simulink model "pdmTransmissionCasing3_new"  (R2020b)
settings: Solver=VariableStepAuto  StartTime=0.0  StopTime=50  FixedStep=0.1  MaxStep=1e-1  RelTol=1e-1  AbsTol=1e-1  EnableMultiTasking=on
PreLoadFcn:
  | ClutchRadius = 100;
  | DampingCoeff = 0.1;
  | SGain = 1;
  | ShaftWear = 0;
  | ToothFaultGain = 0;
  | SDrift = 0;
undefined symbols (not defined in the file or in its folder): sigbuilder_block
libraries: fl_lib x42, nesl_utility x22, sdl_lib x6, commchan3 x2
(part 1 of 2)
CloseFcn:
  | try,close(h1_sdl_transmission_2spd),end
  | clear h1_sdl_transmission_2spd
  | 
  | 
  | clear simlog_sdl_transmission_2spd
  | clear logsout_sdl_transmission_2spd
Description:
  | Two-Speed Transmission
settings Model: FPTRunName=Active  ExtModeAutoUpdateStatusClock=off  Creator=The MathWorks, Inc.  LastModifiedBy=hubert
settings SolverCC: AutoScaleAbsTol=off
settings DataIOCC: MaxDataPoints=10000  SaveFinalState=on  SaveFormat=StructureWithTime  SaveOutput=off  SaveState=on  SaveTime=off  ReturnWorkspaceOutputs=off  LoggingToFile=on  LoggingFileName=out
settings OptimizationCC: ExpressionDepthLimit=2147483647  InitFltsAndDblsToZero=on  LifeSpan=inf
settings DebuggingCC: AlgebraicLoopMsg=none  SaveWithParameterizedLinksMsg=none  UnderspecifiedInitializationDetection=Classic  MergeDetectMultiDrivingBlocksExec=none  CheckExecutionContextPreStartOutputMsg=on  CheckExecutionContextRuntimeOutputMsg=on  SignalResolutionControl=TryResolveAllWithWarning  MultiTaskDSMMsg=warning  MultiTaskCondExecSysMsg=none  FcnCallInpInsideContextMsg=warning  StateNameClashWarn=warning  SFUnexpectedBacktrackingDiag=warning  SFNoUnconditionalDefaultTransitionDiag=warning  SFExecutionAtInitializationDiag=none  ArithmeticOperatorsInVariantConditions=warning
settings HardwareCC: ProdBitPerPointer=32  ProdBitPerSizeT=32  ProdBitPerPtrDiffT=32  ProdLargestAtomicFloat=None  ProdIntDivRoundTo=Undefined  ProdEndianess=Unspecified  ProdWordSize=32  ProdHWDeviceType=32-bit Generic  TargetBitPerLong=64  TargetBitPerPointer=64  TargetBitPerSizeT=64  TargetBitPerPtrDiffT=64  TargetLongLongMode=on  TargetIntDivRoundTo=Zero  TargetEndianess=LittleEndian  TargetWordSize=64  TargetHWDeviceType=MATLAB Host  ProdEqTarget=off
settings ModelReferenceCC: UpdateModelReferenceTargets=IfOutOfDate  PropagateSignalLabelsOutOfModel=off
settings SFSimCC: SimUseLocalCustomCode=off  CustomCodeUndefinedFunction=UseInterfaceOnly
settings RTWCC: RTWUseLocalCustomCode=off
settings CodeAppCC: StateflowObjectComments=on
settings GRTTargetCC: TargetLangStandard=C89/C90 (ANSI)  CombineOutputUpdateFcns=off  GRTInterface=on
settings ConfigComp: CovMetricSettings=dw  CovSaveCumulativeToWorkspaceVar=on  CovSaveSingleToWorkspaceVar=on  CovExternalEMLEnable=off
settings SimscapeCC: SimscapeNormalizeSystem=off  SimscapeLogName=simlog_sdl_transmission_2spd  SimscapeLogDataHistory=10000

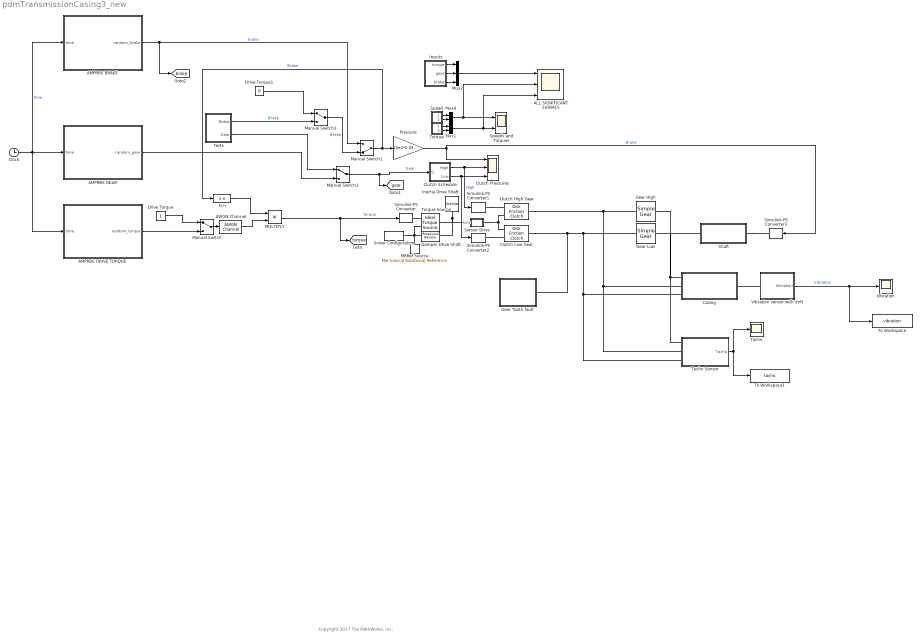
== system pdmTransmissionCasing3_new ==
  note: Copyright 2017 The MathWorks, Inc.
  ALL SIGNIFICANT SIGNALS : Scope  NumInputPorts=3
  AMPRBS BRAKE : Subsystem
  AMPRBS DRIVE TORQUE : Subsystem
  AMPRBS GEAR : Subsystem
  AWGN Channel : commchan3/AWGN Channel  InputProcessing=Columns as channels (frame based)  seed=67  noiseMode=Variance from mask  EbNodB=10  EsNodB=10  SNRdB=10  bitsPerSym=1  Ps=1  Tsym=0.1  variance=0.001
  Casing : Subsystem
  Clock : Clock
  Clutch High Gear : sdl_lib/Clutches/Disk Friction Clutch  geometry_model=1  r_eff=100 mm  d_o=150 mm  d_i=100 mm  nS=4  piston_area=0.001 m^2  unidirectional=0  friction_model=1  mu_w_vector=[ 0 0.1 0.2 0.3 0.4 0.5 1 2 5 10 100 1000 ] rad/s  temperature_TLU=[280.0, 300.0, 320.0] K  mu_static=0.35  mu_static_vector=[0.4, 0.38, 0.36]  mu_coulomb=0.3  mu_coulomb_vector=[ 0.29 0.28 0.26 0.22 0.21 0.2 0.2 0.19 0.19 0.19 0.19 0.19 ]  mu_coulomb_temp_vector=[0.3, 0.28, 0.25]  mu_coulomb_matrix=[0.34, 0.32, 0.3; 0.3, 0.28, 0.25; 0.25, 0.2, 0.15]  mu_interp_method=1  mu_extrap_method=1  d_f=1  w_tol=0.001 rad/s  pressure_min=100 Pa  mu_visc=0 N*m/(rad/s)  initial_state_locked=0  enable_faults=simscape.enum.onoff.off  fault_type=sdl.enum.clutchFault.lock  external_fault=simscape.enum.onoff.off  temporal_fault=simscape.enum.onoff.off  fault_time=5 s  report_fault=simscape.enum.assert.action.none  thermal_mass=25 kJ/K  T_init=300 K
      settings: SourceProductName=Driveline  InternalSimscapePortConfiguration="{\"Bottom\":[],\"Left\":[{\"id\":\"P\",\"label\":\"P\",\"type\":\"input\"},{\"id\":\"B\",\"label\":\"B\",\"type\":\"foundation.mechanical.rotational.rotational\"}],\"Right\":[{\"id\":\"F\",\"label\":\"F\",\"type\":\"foundation.mechanical.rotational.rotational\"}],\"Top\":[]}"
  Clutch Low Gear : sdl_lib/Clutches/Disk Friction Clutch  geometry_model=1  r_eff=ClutchRadius mm  d_o=150 mm  d_i=100 mm  nS=4  piston_area=0.001 m^2  unidirectional=0  friction_model=1  mu_w_vector=[ 0 0.1 0.2 0.3 0.4 0.5 1 2 5 10 100 1000 ] rad/s  temperature_TLU=[280.0, 300.0, 320.0] K  mu_static=0.35  mu_static_vector=[0.4, 0.38, 0.36]  mu_coulomb=0.3  mu_coulomb_vector=[ 0.29 0.28 0.26 0.22 0.21 0.2 0.2 0.19 0.19 0.19 0.19 0.19 ]  mu_coulomb_temp_vector=[0.3, 0.28, 0.25]  mu_coulomb_matrix=[0.34, 0.32, 0.3; 0.3, 0.28, 0.25; 0.25, 0.2, 0.15]  mu_interp_method=1  mu_extrap_method=1  d_f=1  w_tol=0.001 rad/s  pressure_min=100 Pa  mu_visc=0 N*m/(rad/s)  initial_state_locked=0  enable_faults=simscape.enum.onoff.off  fault_type=sdl.enum.clutchFault.lock  external_fault=simscape.enum.onoff.off  temporal_fault=simscape.enum.onoff.off  fault_time=5 s  report_fault=simscape.enum.assert.action.none  thermal_mass=25 kJ/K  T_init=300 K
      settings: SourceProductName=Driveline  InternalSimscapePortConfiguration="{\"Bottom\":[],\"Left\":[{\"id\":\"P\",\"label\":\"P\",\"type\":\"input\"},{\"id\":\"B\",\"label\":\"B\",\"type\":\"foundation.mechanical.rotational.rotational\"}],\"Right\":[{\"id\":\"F\",\"label\":\"F\",\"type\":\"foundation.mechanical.rotational.rotational\"}],\"Top\":[]}"
  Clutch Pressures : Scope  NumInputPorts=3
  Clutch Schedule : Subsystem
  Damper Drive Shaft : fl_lib/Mechanical/Rotational Elements/Rotational Damper  D=DampingCoeff N*m/(rad/s)  w_specify=off  w_priority=High  w=0 rad/s  w_nominal_specify=off  w_nominal_unit=rad/s  w_nominal_value=1  t_specify=off  t_priority=High  t=0 N*m  t_nominal_specify=off  t_nominal_unit=N*m  t_nominal_value=1
      settings: SourceProductName=Foundation Library
  Drive Torque : Constant
  Drive Torque1 : Constant  Value=0
  Fcn : Fcn  Expr=1-u
  Gear High : sdl_lib/Gears/Simple Gear  ratio=2  rotation_direction=3-2*(2)  friction_model=1  mu_visc=[ 0 0 ] N*m/(rad/s)  T_noload=0.1 N*m  T_nom=5 N*m  efficiency_nom=0.8  efficiency=0.8  temperature_TLU=[ 280 300 320 ] K  load_TLU=[ 1 5 10 ] N*m  efficiency_TLU=[ 0.95 0.9 0.85 ]  efficiency_TLU2=[ 0.85 0.8 0.75; 0.95 0.9 0.85; 0.85 0.8 0.7 ]  w_thr=0.01 rad/s  pwr_thr=0.001 W  thermal_mass=50 J/K  enable_faults=simscape.enum.onoff.off  efficiency_fault=0.05  external_fault=simscape.enum.onoff.off  temporal_fault=simscape.enum.onoff.off  fault_time=5 s  fault_angles=pi / 12 rad  report_fault=(1)-1  temperature_specify=off  temperature_priority=High  temperature=300 K  temperature_nominal_specify=off  temperature_nominal_unit=K  temperature_nominal_value=1
      settings: SourceProductName=Driveline
  Gear Low : sdl_lib/Gears/Simple Gear  ratio=5  rotation_direction=3-2*(2)  friction_model=1  mu_visc=[ 0 0 ] N*m/(rad/s)  T_noload=0.1 N*m  T_nom=5 N*m  efficiency_nom=0.8  efficiency=0.8  temperature_TLU=[ 280 300 320 ] K  load_TLU=[ 1 5 10 ] N*m  efficiency_TLU=[ 0.95 0.9 0.85 ]  efficiency_TLU2=[ 0.85 0.8 0.75; 0.95 0.9 0.85; 0.85 0.8 0.7 ]  w_thr=0.01 rad/s  pwr_thr=0.001 W  thermal_mass=50 J/K  enable_faults=simscape.enum.onoff.off  efficiency_fault=0.05  external_fault=simscape.enum.onoff.off  temporal_fault=simscape.enum.onoff.off  fault_time=5 s  fault_angles=pi / 12 rad  report_fault=(1)-1  temperature_specify=off  temperature_priority=High  temperature=300 K  temperature_nominal_specify=off  temperature_nominal_unit=K  temperature_nominal_value=1
      settings: SourceProductName=Driveline
  Gear Tooth fault : Subsystem
  Inertia Drive Shaft : fl_lib/Mechanical/Rotational Elements/Inertia  inertia=1*0.01 kg*m^2  num_ports=foundation.enum.numPorts2.one  w_specify=off  w_priority=High  w=0 rad/s  w_nominal_specify=off  w_nominal_unit=rad/s  w_nominal_value=1  t_specify=off  t_priority=High  t=0 N*m  t_nominal_specify=off  t_nominal_unit=N*m  t_nominal_value=1
      settings: SourceProductName=Foundation Library
  Inputs : Subsystem
  MRRef Source : fl_lib/Mechanical/Rotational Elements/Mechanical Rotational Reference
      settings: SourceProductName=Foundation Library
  MULTIPLY : Product  Inputs=**
  Manual Switch : ManualSwitch
  Manual Switch1 : ManualSwitch  CurrentSetting=0
  Manual Switch2 : ManualSwitch
  Manual Switch3 : ManualSwitch
  Mux1 : Mux  Inputs=2
  Mux2 : Mux  Inputs=3
  Mux4 : Mux  Inputs=2
  Pressure : Gain  Gain=10e2*0.03  SaturateOnIntegerOverflow=on  OutDataTypeStr=Inherit: Same as input  ParamDataTypeStr=Inherit: Same as input
  Sensor Drive : Subsystem
      mask Display: disp('SD')
  Shaft : Subsystem  Variant=on
  Simulink-PS Converter : nesl_utility/Simulink-PS Converter  PhysicalDomain=network_engine_domain  SubClassName=ps_input  LeftPortType=input  RightPortType=output  PseudoPeriodic=off  Frequencies=[]  NoiseDistribution=none  NoiseParameters=[]  Unit=1  AffineConversion=off  FilteringAndDerivatives=zero  SimscapeFilterOrder=1  InputFilterTimeConstant=.001  UdotUserProvided=0
      settings: SourceProductName=Utilities
  Simulink-PS Converter1 : nesl_utility/Simulink-PS Converter  PhysicalDomain=network_engine_domain  SubClassName=ps_input  LeftPortType=input  RightPortType=output  PseudoPeriodic=off  Frequencies=[]  NoiseDistribution=none  NoiseParameters=[]  Unit=Pa  AffineConversion=off  FilteringAndDerivatives=zero  SimscapeFilterOrder=1  InputFilterTimeConstant=.001  UdotUserProvided=0
      settings: SourceProductName=Utilities
  Simulink-PS Converter2 : nesl_utility/Simulink-PS Converter  PhysicalDomain=network_engine_domain  SubClassName=ps_input  LeftPortType=input  RightPortType=output  PseudoPeriodic=off  Frequencies=[]  NoiseDistribution=none  NoiseParameters=[]  Unit=Pa  AffineConversion=off  FilteringAndDerivatives=zero  SimscapeFilterOrder=1  InputFilterTimeConstant=.001  UdotUserProvided=0
      settings: SourceProductName=Utilities
  Simulink-PS Converter3 : nesl_utility/Simulink-PS Converter  PhysicalDomain=network_engine_domain  SubClassName=ps_input  LeftPortType=input  RightPortType=output  PseudoPeriodic=off  Frequencies=[]  NoiseDistribution=none  NoiseParameters=[]  Unit=Pa  AffineConversion=off  FilteringAndDerivatives=zero  SimscapeFilterOrder=1  InputFilterTimeConstant=.001  UdotUserProvided=0
      settings: SourceProductName=Utilities
  Solver Configuration : nesl_utility/Solver Configuration  PhysicalDomain=network_engine_domain  SubClassName=solver  LeftPortType=input  RightPortType=generic  Tones=[]  Harmonics=[]  SimulateNoise=off  Profile=off  UseLocalSampling=off  EnableSwitchedLinearOptims=on  FrequencyDomain=off  UseCCode=off  RelTol=0.001  AbsTol=1e-06  MinStep=1e-09  ToWorkspace=off  RevertToSquareIcSolve=off  NumHomotopyIterations=100  PhasorMode=off  PhasorModeNumHarmonics=1  DoDC=off  ResidualTolerance=1e-9  UseLocalSolver=off  LocalSolverChoice=NE_BACKWARD_EULER_ADVANCER  LocalSolverSampleTime=.001  DoFixedCost=off  MaxNonlinIter=3  MaxModeIter=2  ComputeImpulses=off  ImpulseIterations=2  LinearAlgebra=Sparse  EquationFormulation=NE_TIME_EF  DelaysMemoryBudget=1024  AutomaticFiltering=on  FilteringTimeConstant=0.001  PartitionStorageMethod=AS_NEEDED  PartitionMemoryBudget=1024  PartitionMethod=FAST
      settings: SourceProductName=Utilities
  Speed : Subsystem
  Speeds and Torques : Scope  NumInputPorts=2
  Tacho : Scope
  Tacho Sensor : Subsystem
  Tests : Subsystem  Tag=STV Subsys  LoadFcn=sigbuilder_block('load');  StartFcn=sigbuilder_block('start');  StopFcn=sigbuilder_block('stop');  ClipboardFcn=sigbuilder_block('clipboard');  mask(Sigbuilder block){tuvar=[0:10]}
      mask help: Simulink:masks:SigbuilderBlock_MD
      mask init:
      | if ~strcmp(get_param(bdroot(gcbh),'SimulationStatus'),'stopped') tuvar = sigbuilder_block('maskInit'); end
      settings: CopyFcn=sigbuilder_block('copy');  DeleteFcn=sigbuilder_block('delete');  ModelCloseFcn=sigbuilder_block('modelClose');  PreSaveFcn=sigbuilder_block('preSave');  PauseFcn=sigbuilder_block('pause');  ContinueFcn=sigbuilder_block('continue');  NameChangeFcn=sigbuilder_block('namechange');  OpenFcn=sigbuilder_block('open',[1600.5 1117.5 2958 1396.5 ]);  CloseFcn=sigbuilder_block('close');
      mask Display: plot(0, 0, 100, 100,[2, 2, 32, 32, 2], [68, 8, 8, 68, 68],[32, 2], [38, 38], [32, 19, 2],[53, 60, 44], [32, 17, 17, 2],[16, 16, 31, 31]);txt = getActiveGroup(gcbh);text(2, 100, txt,'verticalAlignment', 'top');
  To Workspace : ToWorkspace  VariableName=vibration  SaveFormat=Timeseries  SampleTime=0.1
  To Workspace1 : ToWorkspace  VariableName=tacho  SaveFormat=Timeseries  SampleTime=0.1
  Torque : Subsystem
  Torque Source : fl_lib/Mechanical/Mechanical Sources/Ideal Torque Source
      settings: SourceProductName=Foundation Library
  Vibration : Scope
  Vibration sensor with drift : Subsystem  VariantControl=Variant < 0
  tag scope: brake=global, gear=global, torque=global
  wires:
  Clutch Schedule/1(High) -> Clutch Pressures/2, Simulink-PS Converter1/1  "High"
  Clutch Schedule/2(Low) -> Clutch Pressures/3, Simulink-PS Converter2/1  "Low"
  Tests/2(Gear) -> Manual Switch2/1
  Manual Switch1/1 -> Fcn/1, Pressure/1  "Brake"
  Speed/1(wD) -> Mux4/1
  Speed/2(wO) -> Mux4/2
  Mux4/1 -> ALL SIGNIFICANT SIGNALS/2, Speeds and Torques/1
  Torque/1(tD) -> Mux1/1
  Torque/2(tO) -> Mux1/2
  Mux1/1 -> ALL SIGNIFICANT SIGNALS/3, Speeds and Torques/2
  Vibration sensor with drift/1(Vibration) -> To Workspace/1, Vibration/1  "Vibration"
  Tacho Sensor/1(Tacho) -> Tacho/1, To Workspace1/1
  Clock/1 -> AMPRBS DRIVE TORQUE/1(time), AMPRBS BRAKE/1(time), AMPRBS GEAR/1(time)  "time"
  AMPRBS BRAKE/1(random_brake) -> [brake], Manual Switch1/1  "brake"
  AMPRBS GEAR/1(random_gear) -> Manual Switch2/2
  Manual Switch2/1 -> [gear], Clutch Schedule/1(G)  "Gear"
  AMPRBS DRIVE TORQUE/1(random_torque) -> Manual Switch/2
  Fcn/1 -> MULTIPLY/1
  Manual Switch/1 -> AWGN Channel/1
  MULTIPLY/1 -> Simulink-PS Converter/1, [torque]  "torque"
  Inputs/1(torque) -> Mux2/1
  Inputs/2(gear) -> Mux2/2
  Inputs/3(brake) -> Mux2/3
  Mux2/1 -> ALL SIGNIFICANT SIGNALS/1
  Drive Torque/1 -> Manual Switch/1
  AWGN Channel/1 -> MULTIPLY/2
  Pressure/1 -> Clutch Pressures/1, Simulink-PS Converter3/1  "Brake"
  Drive Torque1/1 -> Manual Switch3/1
  Tests/1(Brake) -> Manual Switch3/2  "Brake"
  Manual Switch3/1 -> Manual Switch1/2  "Brake"
  connections:
  Clutch High Gear/RConn1 -- Tacho Sensor/LConn2 -- Casing/LConn2 -- Gear High/LConn1
  Simulink-PS Converter1/RConn1 -- Clutch High Gear/LConn1
  Clutch Low Gear/RConn1 -- Gear Tooth fault/LConn1 -- Tacho Sensor/LConn3 -- Casing/LConn3 -- Gear Low/LConn1
  Clutch High Gear/LConn2 -- Clutch Low Gear/LConn2 -- Sensor Drive/RConn1
  Simulink-PS Converter2/RConn1 -- Clutch Low Gear/LConn1
  Inertia Drive Shaft/LConn1 -- Torque Source/LConn1 -- Damper Drive Shaft/LConn1 -- Sensor Drive/LConn1
  Torque Source/RConn2 -- Damper Drive Shaft/RConn1 -- MRRef Source/LConn1 -- Solver Configuration/RConn1
  Torque Source/RConn1 -- Simulink-PS Converter/RConn1
  Vibration sensor with drift/LConn1 -- Casing/RConn1
  Shaft/LConn1 -- Gear Low/RConn1 -- Gear High/RConn1 -- Tacho Sensor/LConn1 -- Casing/LConn1
  Shaft/RConn1 -- Simulink-PS Converter3/RConn1

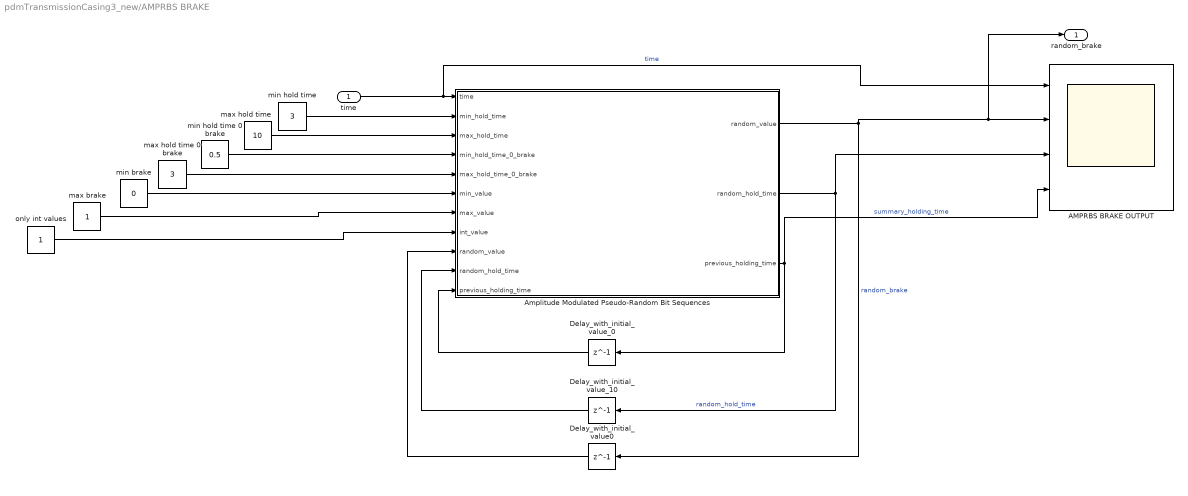
== system pdmTransmissionCasing3_new/AMPRBS BRAKE ==
  time : Inport
  AMPRBS BRAKE OUTPUT : Scope  NumInputPorts=4
  Amplitude Modulated Pseudo-Random Bit Sequences : MATLAB Function  TreatAsAtomicUnit=on  SystemSampleTime=0.1
  Delay_with_initial_value0 : Delay  DelayLength=1  InitialCondition=0
  Delay_with_initial_value_0 : Delay  DelayLength=1  InitialCondition=0
  Delay_with_initial_value_10 : Delay  DelayLength=1  InitialCondition=10
  max brake : Constant
  max hold time : Constant  Value=10
  max hold time 0 brake : Constant  Value=3
  min brake : Constant  Value=0
  min hold time : Constant  Value=3
  min hold time 0 brake : Constant  Value=0.5
  only int values : Constant
  random_brake : Outport
  wires:
  Delay_with_initial_value_10/1 -> Amplitude Modulated Pseudo-Random Bit Sequences/10("random_hold_time ")
  Amplitude Modulated Pseudo-Random Bit Sequences/1(random_value) -> random_brake/1, AMPRBS BRAKE OUTPUT/2, Delay_with_initial_value0/1  "random_brake"
  time/1 -> AMPRBS BRAKE OUTPUT/1, Amplitude Modulated Pseudo-Random Bit Sequences/1(time)  "time"
  Amplitude Modulated Pseudo-Random Bit Sequences/3(previous_holding_time) -> AMPRBS BRAKE OUTPUT/4, Delay_with_initial_value_0/1  "summary_holding_time"
  Delay_with_initial_value_0/1 -> Amplitude Modulated Pseudo-Random Bit Sequences/11("previous_holding_time ")
  Amplitude Modulated Pseudo-Random Bit Sequences/2(random_hold_time) -> AMPRBS BRAKE OUTPUT/3, Delay_with_initial_value_10/1  "random_hold_time"
  Delay_with_initial_value0/1 -> Amplitude Modulated Pseudo-Random Bit Sequences/9("random_value ")
  min brake/1 -> Amplitude Modulated Pseudo-Random Bit Sequences/6(min_value)
  max brake/1 -> Amplitude Modulated Pseudo-Random Bit Sequences/7(max_value)
  min hold time/1 -> Amplitude Modulated Pseudo-Random Bit Sequences/2(min_hold_time)
  max hold time/1 -> Amplitude Modulated Pseudo-Random Bit Sequences/3(max_hold_time)
  only int values/1 -> Amplitude Modulated Pseudo-Random Bit Sequences/8(int_value)
  max hold time 0 brake/1 -> Amplitude Modulated Pseudo-Random Bit Sequences/5(max_hold_time_0_brake)
  min hold time 0 brake/1 -> Amplitude Modulated Pseudo-Random Bit Sequences/4(min_hold_time_0_brake)

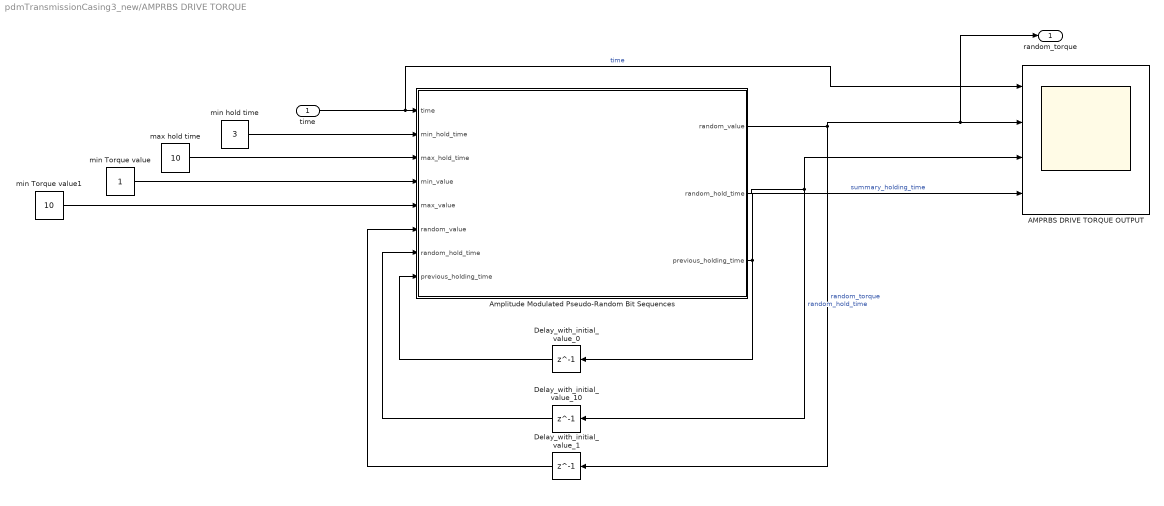
== system pdmTransmissionCasing3_new/AMPRBS DRIVE TORQUE ==
  time : Inport
  AMPRBS DRIVE TORQUE OUTPUT : Scope  NumInputPorts=4
  Amplitude Modulated Pseudo-Random Bit Sequences : MATLAB Function  TreatAsAtomicUnit=on  SystemSampleTime=0.1
  Delay_with_initial_value_0 : Delay  DelayLength=1  InitialCondition=0
  Delay_with_initial_value_1 : Delay  DelayLength=1  InitialCondition=1
  Delay_with_initial_value_10 : Delay  DelayLength=1  InitialCondition=10
  max hold time : Constant  Value=10
  min Torque value : Constant
  min Torque value1 : Constant  Value=10
  min hold time : Constant  Value=3
  random_torque : Outport
  wires:
  Delay_with_initial_value_10/1 -> Amplitude Modulated Pseudo-Random Bit Sequences/7("random_hold_time ")
  Amplitude Modulated Pseudo-Random Bit Sequences/1(random_value) -> random_torque/1, AMPRBS DRIVE TORQUE OUTPUT/2, Delay_with_initial_value_1/1  "random_torque"
  time/1 -> AMPRBS DRIVE TORQUE OUTPUT/1, Amplitude Modulated Pseudo-Random Bit Sequences/1(time)  "time"
  Amplitude Modulated Pseudo-Random Bit Sequences/3(previous_holding_time) -> AMPRBS DRIVE TORQUE OUTPUT/4, Delay_with_initial_value_0/1  "summary_holding_time"
  Delay_with_initial_value_0/1 -> Amplitude Modulated Pseudo-Random Bit Sequences/8("previous_holding_time ")
  Amplitude Modulated Pseudo-Random Bit Sequences/2(random_hold_time) -> AMPRBS DRIVE TORQUE OUTPUT/3, Delay_with_initial_value_10/1  "random_hold_time"
  Delay_with_initial_value_1/1 -> Amplitude Modulated Pseudo-Random Bit Sequences/6("random_value ")
  min Torque value/1 -> Amplitude Modulated Pseudo-Random Bit Sequences/4(min_value)
  min Torque value1/1 -> Amplitude Modulated Pseudo-Random Bit Sequences/5(max_value)
  min hold time/1 -> Amplitude Modulated Pseudo-Random Bit Sequences/2(min_hold_time)
  max hold time/1 -> Amplitude Modulated Pseudo-Random Bit Sequences/3(max_hold_time)

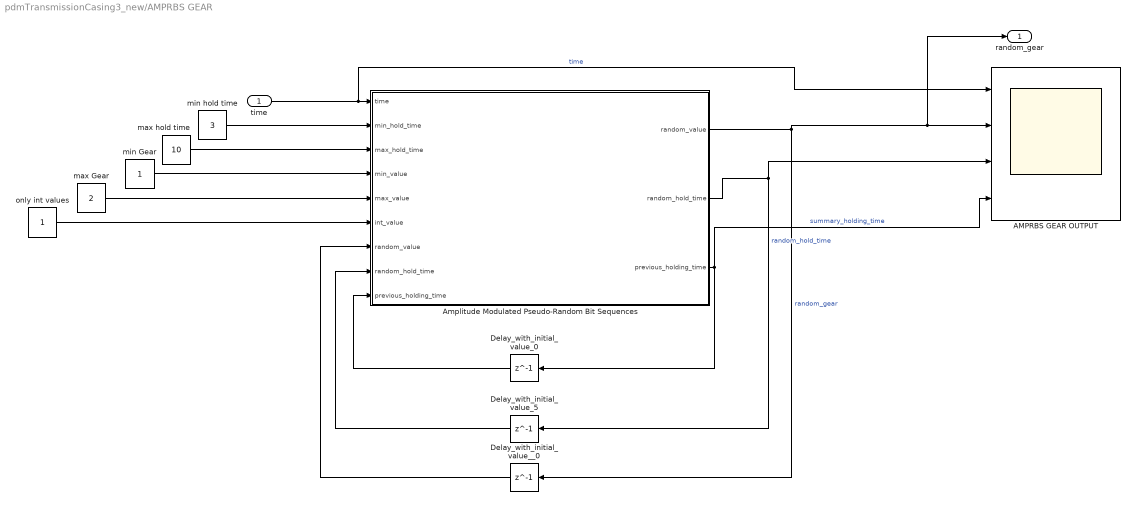
== system pdmTransmissionCasing3_new/AMPRBS GEAR ==
  time : Inport
  AMPRBS GEAR OUTPUT : Scope  NumInputPorts=4
  Amplitude Modulated Pseudo-Random Bit Sequences : MATLAB Function  TreatAsAtomicUnit=on  SystemSampleTime=0.1
  Delay_with_initial_value_0 : Delay  DelayLength=1  InitialCondition=0
  Delay_with_initial_value_5 : Delay  DelayLength=1  InitialCondition=5
  Delay_with_initial_value__0 : Delay  DelayLength=1  InitialCondition=0
  max Gear : Constant  Value=2
  max hold time : Constant  Value=10
  min Gear : Constant
  min hold time : Constant  Value=3
  only int values : Constant
  random_gear : Outport
  wires:
  Delay_with_initial_value_5/1 -> Amplitude Modulated Pseudo-Random Bit Sequences/8("random_hold_time ")
  Amplitude Modulated Pseudo-Random Bit Sequences/1(random_value) -> random_gear/1, AMPRBS GEAR OUTPUT/2, Delay_with_initial_value__0/1  "random_gear"
  time/1 -> AMPRBS GEAR OUTPUT/1, Amplitude Modulated Pseudo-Random Bit Sequences/1(time)  "time"
  Amplitude Modulated Pseudo-Random Bit Sequences/3(previous_holding_time) -> AMPRBS GEAR OUTPUT/4, Delay_with_initial_value_0/1  "summary_holding_time"
  Delay_with_initial_value_0/1 -> Amplitude Modulated Pseudo-Random Bit Sequences/9("previous_holding_time ")
  Amplitude Modulated Pseudo-Random Bit Sequences/2(random_hold_time) -> Delay_with_initial_value_5/1, AMPRBS GEAR OUTPUT/3  "random_hold_time"
  Delay_with_initial_value__0/1 -> Amplitude Modulated Pseudo-Random Bit Sequences/7("random_value ")
  min Gear/1 -> Amplitude Modulated Pseudo-Random Bit Sequences/4(min_value)
  max Gear/1 -> Amplitude Modulated Pseudo-Random Bit Sequences/5(max_value)
  min hold time/1 -> Amplitude Modulated Pseudo-Random Bit Sequences/2(min_hold_time)
  max hold time/1 -> Amplitude Modulated Pseudo-Random Bit Sequences/3(max_hold_time)
  only int values/1 -> Amplitude Modulated Pseudo-Random Bit Sequences/6(int_value)

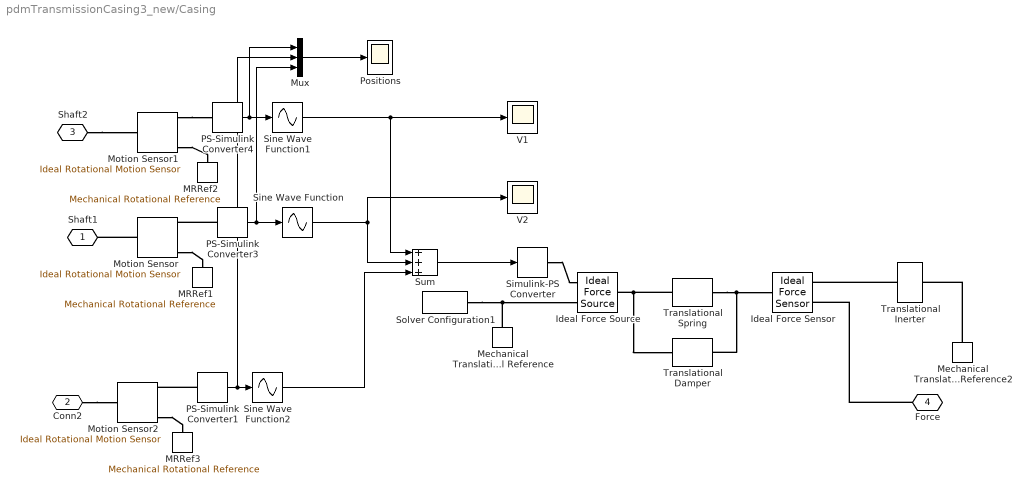
== system pdmTransmissionCasing3_new/Casing ==
  Ideal Force Sensor : fl_lib/Mechanical/Mechanical Sensors/Ideal Force Sensor
      settings: SourceProductName=Foundation Library
  Ideal Force Source : fl_lib/Mechanical/Mechanical Sources/Ideal Force Source
      settings: SourceProductName=Foundation Library
  MRRef1 : fl_lib/Mechanical/Rotational Elements/Mechanical Rotational Reference
      settings: SourceProductName=Foundation Library
  MRRef2 : fl_lib/Mechanical/Rotational Elements/Mechanical Rotational Reference
      settings: SourceProductName=Foundation Library
  MRRef3 : fl_lib/Mechanical/Rotational Elements/Mechanical Rotational Reference
      settings: SourceProductName=Foundation Library
  Mechanical Translational Reference : fl_lib/Mechanical/Translational Elements/Mechanical Translational Reference
      settings: SourceProductName=Foundation Library
  Mechanical Translational Reference2 : fl_lib/Mechanical/Translational Elements/Mechanical Translational Reference
      settings: SourceProductName=Foundation Library
  Motion Sensor : fl_lib/Mechanical/Mechanical Sensors/Ideal Rotational Motion Sensor  wrap_angle=simscape.enum.onoff.off  offset=0 rad
      settings: SourceProductName=Foundation Library
  Motion Sensor1 : fl_lib/Mechanical/Mechanical Sensors/Ideal Rotational Motion Sensor  wrap_angle=simscape.enum.onoff.off  offset=0 rad
      settings: SourceProductName=Foundation Library
  Motion Sensor2 : fl_lib/Mechanical/Mechanical Sensors/Ideal Rotational Motion Sensor  wrap_angle=simscape.enum.onoff.off  offset=0 rad
      settings: SourceProductName=Foundation Library
  Mux : Mux  Inputs=3
  PS-Simulink Converter1 : nesl_utility/PS-Simulink Converter  PhysicalDomain=network_engine_domain  SubClassName=ps_output  LeftPortType=input  RightPortType=output  PseudoPeriodic=off  Frequencies=[]  Unit=rad  AffineConversion=off
      settings: SourceProductName=Utilities
  PS-Simulink Converter3 : nesl_utility/PS-Simulink Converter  PhysicalDomain=network_engine_domain  SubClassName=ps_output  LeftPortType=input  RightPortType=output  PseudoPeriodic=off  Frequencies=[]  Unit=rad  AffineConversion=off
      settings: SourceProductName=Utilities
  PS-Simulink Converter4 : nesl_utility/PS-Simulink Converter  PhysicalDomain=network_engine_domain  SubClassName=ps_output  LeftPortType=input  RightPortType=output  PseudoPeriodic=off  Frequencies=[]  Unit=rad  AffineConversion=off
      settings: SourceProductName=Utilities
  Positions : Scope
  Simulink-PS Converter : nesl_utility/Simulink-PS Converter  PhysicalDomain=network_engine_domain  SubClassName=ps_input  LeftPortType=input  RightPortType=output  PseudoPeriodic=off  Frequencies=[]  NoiseDistribution=none  NoiseParameters=[]  Unit=N  AffineConversion=off  FilteringAndDerivatives=zero  SimscapeFilterOrder=1  InputFilterTimeConstant=0.001  UdotUserProvided=1
      settings: SourceProductName=Utilities
  Sine Wave Function : Sin  TimeSource=Use external signal  SampleTime=0
  Sine Wave Function1 : Sin  TimeSource=Use external signal  SampleTime=0
  Sine Wave Function2 : Sin  TimeSource=Use external signal  SampleTime=0
  Solver Configuration1 : nesl_utility/Solver Configuration  PhysicalDomain=network_engine_domain  SubClassName=solver  LeftPortType=input  RightPortType=generic  Tones=[]  Harmonics=[]  SimulateNoise=off  Profile=off  UseLocalSampling=off  EnableSwitchedLinearOptims=on  FrequencyDomain=off  UseCCode=off  RelTol=0.001  AbsTol=1e-06  MinStep=1e-09  ToWorkspace=off  RevertToSquareIcSolve=off  NumHomotopyIterations=100  PhasorMode=off  PhasorModeNumHarmonics=1  DoDC=off  ResidualTolerance=1e-9  UseLocalSolver=off  LocalSolverChoice=NE_TRAPEZOIDAL_ADVANCER  LocalSolverSampleTime=0.0001  DoFixedCost=off  MaxNonlinIter=3  MaxModeIter=2  ComputeImpulses=off  ImpulseIterations=2  LinearAlgebra=Sparse  EquationFormulation=NE_TIME_EF  DelaysMemoryBudget=1024  AutomaticFiltering=on  FilteringTimeConstant=0.001  PartitionStorageMethod=AS_NEEDED  PartitionMemoryBudget=1024  PartitionMethod=FAST
      settings: SourceProductName=Utilities
  Sum : Sum  Inputs=+++
  Translational Inerter : fl_lib/Mechanical/Translational Elements/Translational Inerter  B=1 kg  v_specify=off  v_priority=High  v=0 m/s  v_nominal_specify=off  v_nominal_unit=m/s  v_nominal_value=1  f_specify=off  f_priority=None  f=0 N  f_nominal_specify=off  f_nominal_unit=N  f_nominal_value=1
      settings: SourceProductName=Foundation Library  InternalSimscapePortConfiguration="{\"Bottom\":[],\"Left\":[{\"id\":\"R\",\"label\":\"R\",\"type\":\"foundation.mechanical.translational.translational\"}],\"Right\":[{\"id\":\"C\",\"label\":\"C\",\"type\":\"foundation.mechanical.translational.translational\"}],\"Top\":[]}"
  Translational Damper : fl_lib/Mechanical/Translational Elements/Translational Damper  D=100 N/(m/s)  v_specify=off  v_priority=None  v=0 m/s  v_nominal_specify=off  v_nominal_unit=m/s  v_nominal_value=1  f_specify=off  f_priority=None  f=0 N  f_nominal_specify=off  f_nominal_unit=N  f_nominal_value=1
      settings: SourceProductName=Foundation Library
  Translational Spring : fl_lib/Mechanical/Translational Elements/Translational Spring  spr_rate=1000 N/m  v_specify=off  v_priority=None  v=0 m/s  v_nominal_specify=off  v_nominal_unit=m/s  v_nominal_value=1  f_specify=off  f_priority=None  f=0 N  f_nominal_specify=off  f_nominal_unit=N  f_nominal_value=1  x_specify=off  x_priority=High  x=0 m  x_nominal_specify=off  x_nominal_unit=m  x_nominal_value=1
      settings: SourceProductName=Foundation Library
  V1 : Scope
  V2 : Scope
  Shaft1 : PMIOPort  Side=Left
  Conn2 : PMIOPort  Port=2  Side=Left
  Shaft2 : PMIOPort  Port=3  Side=Left
  Force : PMIOPort  Port=4  Side=Right
  wires:
  Sum/1 -> Simulink-PS Converter/1
  PS-Simulink Converter4/1 -> Mux/1, Sine Wave Function1/1
  PS-Simulink Converter3/1 -> Mux/3, Sine Wave Function/1
  Sine Wave Function/1 -> V2/1, Sum/2
  Sine Wave Function1/1 -> V1/1, Sum/1
  Mux/1 -> Positions/1
  PS-Simulink Converter1/1 -> Mux/2, Sine Wave Function2/1
  Sine Wave Function2/1 -> Sum/3
  connections:
  Simulink-PS Converter/RConn1 -- Ideal Force Source/RConn1
  Motion Sensor/LConn1 -- Shaft1/RConn1
  Translational Inerter/LConn1 -- Ideal Force Sensor/RConn1
  Motion Sensor1/RConn3 -- PS-Simulink Converter4/LConn1
  Motion Sensor1/RConn1 -- MRRef2/LConn1
  Mechanical Translational Reference2/LConn1 -- Translational Inerter/RConn1
  Force/RConn1 -- Ideal Force Sensor/RConn2
  Shaft2/RConn1 -- Motion Sensor1/LConn1
  Solver Configuration1/RConn1 -- Mechanical Translational Reference/LConn1 -- Ideal Force Source/RConn2
  Translational Spring/RConn1 -- Ideal Force Sensor/LConn1 -- Translational Damper/RConn1
  Translational Spring/LConn1 -- Translational Damper/LConn1 -- Ideal Force Source/LConn1
  PS-Simulink Converter3/LConn1 -- Motion Sensor/RConn3
  Motion Sensor/RConn1 -- MRRef1/LConn1
  PS-Simulink Converter1/LConn1 -- Motion Sensor2/RConn3
  Conn2/RConn1 -- Motion Sensor2/LConn1
  Motion Sensor2/RConn1 -- MRRef3/LConn1

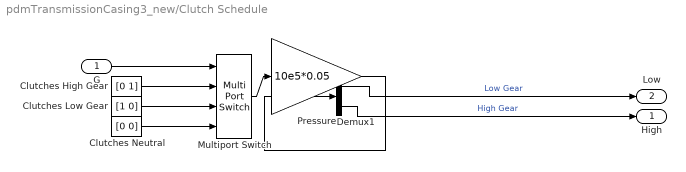
== system pdmTransmissionCasing3_new/Clutch Schedule ==
  G : Inport
  Clutches High Gear : Constant  Value=[0 1]
  Clutches Low Gear : Constant  Value=[1 0]
  Clutches Neutral : Constant  Value=[0 0]
  Demux1 : Demux  Outputs=2
  Multiport Switch : MultiPortSwitch  DataPortOrder=Specify indices  DataPortIndices={2,1,0}
  Pressure : Gain  Gain=10e5*0.05  SaturateOnIntegerOverflow=on  OutDataTypeStr=Inherit: Same as input  ParamDataTypeStr=Inherit: Same as input
  High : Outport  VectorParamsAs1DForOutWhenUnconnected=off
  Low : Outport  Port=2  VectorParamsAs1DForOutWhenUnconnected=off
  wires:
  G/1 -> Multiport Switch/1
  Clutches High Gear/1 -> Multiport Switch/2
  Clutches Low Gear/1 -> Multiport Switch/3
  Clutches Neutral/1 -> Multiport Switch/4
  Multiport Switch/1 -> Pressure/1
  Demux1/2 -> High/1  "High Gear"
  Demux1/1 -> Low/1  "Low Gear"
  Pressure/1 -> Demux1/1

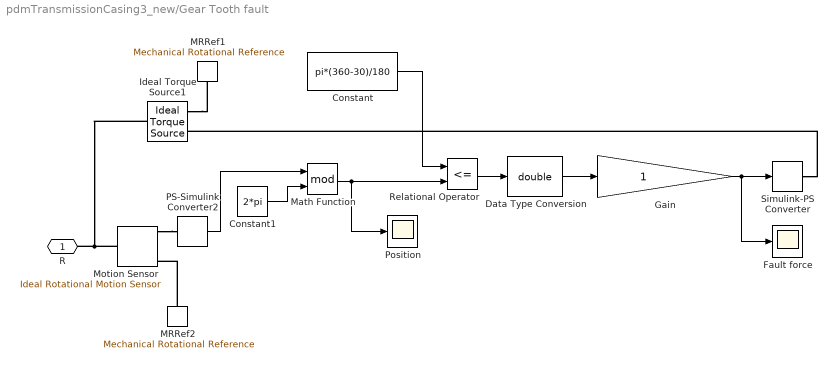
== system pdmTransmissionCasing3_new/Gear Tooth fault ==
  Constant : Constant  Value=pi*(360-30)/180
  Constant1 : Constant  Value=2*pi
  Data Type Conversion : DataTypeConversion  OutDataTypeStr=double
  Fault force : Scope
  Gain : Gain
  Ideal Torque Source1 : fl_lib/Mechanical/Mechanical Sources/Ideal Torque Source
      settings: SourceProductName=Foundation Library
  MRRef1 : fl_lib/Mechanical/Rotational Elements/Mechanical Rotational Reference
      settings: SourceProductName=Foundation Library
  MRRef2 : fl_lib/Mechanical/Rotational Elements/Mechanical Rotational Reference
      settings: SourceProductName=Foundation Library
  Math Function : Math  Operator=mod  SignedPower=on  SaturateOnIntegerOverflow=on
  Motion Sensor : fl_lib/Mechanical/Mechanical Sensors/Ideal Rotational Motion Sensor  wrap_angle=simscape.enum.onoff.off  offset=0 rad
      settings: SourceProductName=Foundation Library
  PS-Simulink Converter2 : nesl_utility/PS-Simulink Converter  PhysicalDomain=network_engine_domain  SubClassName=ps_output  LeftPortType=input  RightPortType=output  PseudoPeriodic=off  Frequencies=[]  Unit=rad  AffineConversion=off
      settings: SourceProductName=Utilities
  Position : Scope
  Relational Operator : RelationalOperator  Operator=<=  OutDataTypeStr=boolean  RndMeth=Simplest
  Simulink-PS Converter : nesl_utility/Simulink-PS Converter  PhysicalDomain=network_engine_domain  SubClassName=ps_input  LeftPortType=input  RightPortType=output  PseudoPeriodic=off  Frequencies=[]  NoiseDistribution=none  NoiseParameters=[]  Unit=1  AffineConversion=off  FilteringAndDerivatives=zero  SimscapeFilterOrder=1  InputFilterTimeConstant=0.001  UdotUserProvided=1
      settings: SourceProductName=Utilities
  R : PMIOPort  Side=Left
  wires:
  Gain/1 -> Fault force/1, Simulink-PS Converter/1
  Constant/1 -> Relational Operator/1
  Relational Operator/1 -> Data Type Conversion/1
  Data Type Conversion/1 -> Gain/1
  Constant1/1 -> Math Function/2
  Math Function/1 -> Relational Operator/2, Position/1
  PS-Simulink Converter2/1 -> Math Function/1
  connections:
  MRRef2/LConn1 -- Motion Sensor/RConn1
  Motion Sensor/RConn3 -- PS-Simulink Converter2/LConn1
  Motion Sensor/LConn1 -- Ideal Torque Source1/LConn1 -- R/RConn1
  Simulink-PS Converter/RConn1 -- Ideal Torque Source1/RConn1
  Ideal Torque Source1/RConn2 -- MRRef1/LConn1

== system pdmTransmissionCasing3_new/Inputs ==
  torque : Outport  VectorParamsAs1DForOutWhenUnconnected=off
  gear : Outport  Port=2  VectorParamsAs1DForOutWhenUnconnected=off
  brake : Outport  Port=3  VectorParamsAs1DForOutWhenUnconnected=off
  wires:
  [torque] -> torque/1  "torque"
  [gear] -> gear/1  "gear"
  [brake] -> brake/1  "brake"

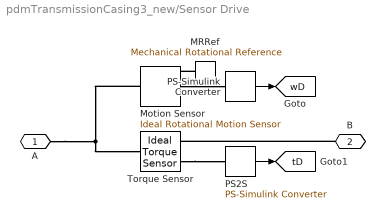
== system pdmTransmissionCasing3_new/Sensor Drive ==
  MRRef : fl_lib/Mechanical/Rotational Elements/Mechanical Rotational Reference
      settings: SourceProductName=Foundation Library
  Motion Sensor : fl_lib/Mechanical/Mechanical Sensors/Ideal Rotational Motion Sensor  wrap_angle=simscape.enum.onoff.off  offset=0 rad
      settings: SourceProductName=Foundation Library
  PS-Simulink Converter : nesl_utility/PS-Simulink Converter  PhysicalDomain=network_engine_domain  SubClassName=ps_output  LeftPortType=input  RightPortType=output  PseudoPeriodic=off  Frequencies=[]  Unit=rpm  AffineConversion=off
      settings: SourceProductName=Utilities
  PS2S : nesl_utility/PS-Simulink Converter  PhysicalDomain=network_engine_domain  SubClassName=ps_output  LeftPortType=input  RightPortType=output  PseudoPeriodic=off  Frequencies=[]  Unit=1  AffineConversion=off
      settings: SourceProductName=Utilities
  Torque Sensor : fl_lib/Mechanical/Mechanical Sensors/Ideal Torque Sensor
      settings: SourceProductName=Foundation Library
  A : PMIOPort  Side=Left
  B : PMIOPort  Port=2  Side=Right
  tag scope: tD=global, wD=global
  wires:
  PS2S/1 -> [tD]
  PS-Simulink Converter/1 -> [wD]
  connections:
  B/RConn1 -- Torque Sensor/RConn1
  A/RConn1 -- Motion Sensor/LConn1 -- Torque Sensor/LConn1
  Torque Sensor/RConn2 -- PS2S/LConn1
  MRRef/LConn1 -- Motion Sensor/RConn1
  Motion Sensor/RConn2 -- PS-Simulink Converter/LConn1

== system pdmTransmissionCasing3_new/Shaft ==
  note: 1) Add Subsystem or Model blocks as valid variant choices.
      | 2) You cannot connect blocks at this level. At simulation, connectivity is automatically
      | determined, based on the active variant and port name matching.
  Output Shaft : Subsystem  VariantControl=ShaftWear >=0
  Worn Output Shaft : Subsystem  VariantControl=ShaftWear < 0
  Shaft : PMIOPort  Side=Left
  Brake : PMIOPort  Port=2  Side=Right

== system pdmTransmissionCasing3_new/Speed ==
  Gain : Gain  Gain=-1
  wD : Outport  VectorParamsAs1DForOutWhenUnconnected=off
  wO : Outport  Port=2  VectorParamsAs1DForOutWhenUnconnected=off
  wires:
  [wD] -> wD/1  "Drive"
  [wO] -> Gain/1
  Gain/1 -> wO/1  "Output"

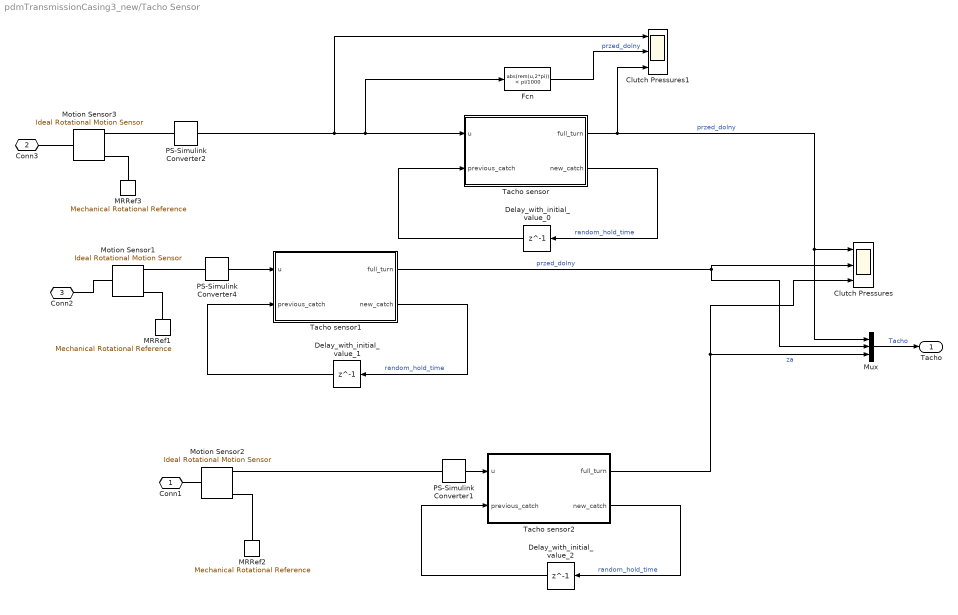
== system pdmTransmissionCasing3_new/Tacho Sensor ==
  Clutch Pressures : Scope  NumInputPorts=3
  Clutch Pressures1 : Scope  NumInputPorts=3
  Delay_with_initial_value_0 : Delay  DelayLength=1  InitialCondition=0
  Delay_with_initial_value_1 : Delay  DelayLength=1  InitialCondition=0
  Delay_with_initial_value_2 : Delay  DelayLength=1  InitialCondition=0
  Fcn : Fcn  Expr=abs(rem(u,2*pi)) < pi/1000
  MRRef1 : fl_lib/Mechanical/Rotational Elements/Mechanical Rotational Reference
      settings: SourceProductName=Foundation Library
  MRRef2 : fl_lib/Mechanical/Rotational Elements/Mechanical Rotational Reference
      settings: SourceProductName=Foundation Library
  MRRef3 : fl_lib/Mechanical/Rotational Elements/Mechanical Rotational Reference
      settings: SourceProductName=Foundation Library
  Motion Sensor1 : fl_lib/Mechanical/Mechanical Sensors/Ideal Rotational Motion Sensor  wrap_angle=simscape.enum.onoff.off  offset=0 rad
      settings: SourceProductName=Foundation Library
  Motion Sensor2 : fl_lib/Mechanical/Mechanical Sensors/Ideal Rotational Motion Sensor  wrap_angle=simscape.enum.onoff.off  offset=0 rad
      settings: SourceProductName=Foundation Library
  Motion Sensor3 : fl_lib/Mechanical/Mechanical Sensors/Ideal Rotational Motion Sensor  wrap_angle=simscape.enum.onoff.off  offset=0 rad
      settings: SourceProductName=Foundation Library
  Mux : Mux  Inputs=3
  PS-Simulink Converter1 : nesl_utility/PS-Simulink Converter  PhysicalDomain=network_engine_domain  SubClassName=ps_output  LeftPortType=input  RightPortType=output  PseudoPeriodic=off  Frequencies=[]  Unit=rad  AffineConversion=off
      settings: SourceProductName=Utilities
  PS-Simulink Converter2 : nesl_utility/PS-Simulink Converter  PhysicalDomain=network_engine_domain  SubClassName=ps_output  LeftPortType=input  RightPortType=output  PseudoPeriodic=off  Frequencies=[]  Unit=rad  AffineConversion=off
      settings: SourceProductName=Utilities
  PS-Simulink Converter4 : nesl_utility/PS-Simulink Converter  PhysicalDomain=network_engine_domain  SubClassName=ps_output  LeftPortType=input  RightPortType=output  PseudoPeriodic=off  Frequencies=[]  Unit=rad  AffineConversion=off
      settings: SourceProductName=Utilities
  Tacho sensor : MATLAB Function  TreatAsAtomicUnit=on  SystemSampleTime=0.1
  Tacho sensor1 : MATLAB Function  TreatAsAtomicUnit=on  SystemSampleTime=0.1
  Tacho sensor2 : MATLAB Function  TreatAsAtomicUnit=on  SystemSampleTime=0.1
  Conn1 : PMIOPort  Side=Left
  Conn3 : PMIOPort  Port=2  Side=Left
  Conn2 : PMIOPort  Port=3  Side=Left
  Tacho : Outport  VectorParamsAs1DForOutWhenUnconnected=off
  wires:
  PS-Simulink Converter1/1 -> Tacho sensor2/1(u)
  PS-Simulink Converter4/1 -> Tacho sensor1/1(u)
  Mux/1 -> Tacho/1  "Tacho"
  PS-Simulink Converter2/1 -> Fcn/1, Tacho sensor/1(u), Clutch Pressures1/1
  Tacho sensor/1(full_turn) -> Mux/1, Clutch Pressures/1, Clutch Pressures1/3  "przed_dolny"
  Tacho sensor2/1(full_turn) -> Clutch Pressures/3, Mux/3  "za"
  Tacho sensor1/1(full_turn) -> Clutch Pressures/2, Mux/2  "przed_dolny"
  Delay_with_initial_value_0/1 -> Tacho sensor/2(previous_catch)
  Tacho sensor/2(new_catch) -> Delay_with_initial_value_0/1  "random_hold_time"
  Fcn/1 -> Clutch Pressures1/2  "przed_dolny"
  Delay_with_initial_value_1/1 -> Tacho sensor1/2(previous_catch)
  Tacho sensor1/2(new_catch) -> Delay_with_initial_value_1/1  "random_hold_time"
  Delay_with_initial_value_2/1 -> Tacho sensor2/2(previous_catch)
  Tacho sensor2/2(new_catch) -> Delay_with_initial_value_2/1  "random_hold_time"
  connections:
  Motion Sensor2/RConn3 -- PS-Simulink Converter1/LConn1
  PS-Simulink Converter4/LConn1 -- Motion Sensor1/RConn3
  Motion Sensor2/RConn1 -- MRRef2/LConn1
  Motion Sensor1/RConn1 -- MRRef1/LConn1
  Conn2/RConn1 -- Motion Sensor1/LConn1
  Conn1/RConn1 -- Motion Sensor2/LConn1
  Conn3/RConn1 -- Motion Sensor3/LConn1
  PS-Simulink Converter2/LConn1 -- Motion Sensor3/RConn3
  Motion Sensor3/RConn1 -- MRRef3/LConn1

== system pdmTransmissionCasing3_new/Tests ==
  Demux : Demux  Tag=STV Demux  Outputs=2
      settings: DisplayOption=none
  FromWs : FromWorkspace  Tag=STV FromWs  VariableName=tuvar
      SigBuilderData=|
      | common.afterFinalStr = 'Extrapolate'
      | common.sampleTime = 0
      | dataSet(1).timeRange = [0 50]
      | dataSet(1).name = 'T1'
      | dataSet(2).timeRange = [0 50]
      | dataSet(2).name = 'T2'
      | dataSet(3).timeRange = [0 50]
      | dataSet(3).name = 'T3'
      | sbobj.Groups(1).Name = 'T1'
      | sbobj.Groups(1).Signals(1).Name = 'Brake'
      | sbobj.Groups(1).Signals(1).XData = [0 15 15 20 20 35 35 40 40 50]
      | sbobj.Groups(1).Signals(1).YData = [0 0 1 1 0 0 1 1 0 0]
      | sbobj.Groups(1).Signals(2).Name = 'Gear'
      | sbobj.Groups(1).Signals(2).XData = [0 5 5 10 10 30 30 40 50]
      | sbobj.Groups(1).Signals(2).YData = [0 0 1 1 2 2 0 0 0]
      | sbobj.Groups(1).TimeRange = [0 50]
      | sbobj.Groups(2).Name = 'T2'
      | sbobj.Groups(2).Signals(1).Name = 'Brake'
      | sbobj.Groups(2).Signals(1).XData = [0 15 20 20 35 35 40 50]
      | sbobj.Groups(2).Signals(1).YData = [0 0 0 0.004 0.004 1 1 1]
      | sbobj.Groups(2).Signals(2).Name = 'Gear'
      | sbobj.Groups(2).Signals(2).XData = [0 5 5 10 40 40 50]
      | sbobj.Groups(2).Signals(2).YData = [0 0 1 1 1 0 0]
      | sbobj.Groups(2).TimeRange = [0 50]
      | sbobj.Groups(3).Name = 'T3'
      | sbobj.Groups(3).Signals(1).Name = 'Brake'
      | sbobj.Groups(3).Signals(1).XData = [0 15 20 35 40 50]
      | sbobj.Groups(3).Signals(1).YData = [0 0 0 0 0 0]
      | sbobj.Groups(3).Signals(2).Name = 'Gear'
      | sbobj.Groups(3).Signals(2).XData = [0 5 5 10 10 40 40 50]
      | sbobj.Groups(3).Signals(2).YData = [0 0 1 1 2 2 0 0]
      | sbobj.Groups(3).TimeRange = [0 50]
  Brake : Outport  Tag=STV Outport  VectorParamsAs1DForOutWhenUnconnected=off
  Gear : Outport  Tag=STV Outport  Port=2  VectorParamsAs1DForOutWhenUnconnected=off
  wires:
  Demux/1 -> Brake/1
  FromWs/1 -> Demux/1
  Demux/2 -> Gear/1

== system pdmTransmissionCasing3_new/Torque ==
  tD : Outport  VectorParamsAs1DForOutWhenUnconnected=off
  tO : Outport  Port=2  VectorParamsAs1DForOutWhenUnconnected=off
  wires:
  [tD] -> tD/1  "Drive"
  [tO] -> tO/1  "Output"

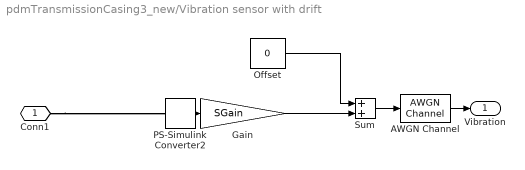
== system pdmTransmissionCasing3_new/Vibration sensor with drift ==
  AWGN Channel : commchan3/AWGN Channel  InputProcessing=Columns as channels (frame based)  seed=67  noiseMode=Variance from mask  EbNodB=10  EsNodB=10  SNRdB=10  bitsPerSym=1  Ps=1  Tsym=0.1  variance=0.001
  Gain : Gain  Gain=SGain
  Offset : Constant  Value=0
  PS-Simulink Converter2 : nesl_utility/PS-Simulink Converter  PhysicalDomain=network_engine_domain  SubClassName=ps_output  LeftPortType=input  RightPortType=output  PseudoPeriodic=off  Frequencies=[]  Unit=N  AffineConversion=off
      settings: SourceProductName=Utilities
  Sum : Sum
  Conn1 : PMIOPort  Side=Left
  Vibration : Outport  VectorParamsAs1DForOutWhenUnconnected=off
  wires:
  Sum/1 -> AWGN Channel/1
  PS-Simulink Converter2/1 -> Gain/1
  Offset/1 -> Sum/1
  Gain/1 -> Sum/2
  AWGN Channel/1 -> Vibration/1
  connections:
  Conn1/RConn1 -- PS-Simulink Converter2/LConn1

== system pdmTransmissionCasing3_new/Shaft/Output Shaft ==
  Clutch Brake : sdl_lib/Clutches/Disk Friction Clutch  geometry_model=1  r_eff=100 mm  d_o=150 mm  d_i=100 mm  nS=4  piston_area=0.001 m^2  unidirectional=0  friction_model=1  mu_w_vector=[ 0 0.1 0.2 0.3 0.4 0.5 1 2 5 10 100 1000 ] rad/s  temperature_TLU=[280.0, 300.0, 320.0] K  mu_static=0.35  mu_static_vector=[0.4, 0.38, 0.36]  mu_coulomb=0.3  mu_coulomb_vector=[ 0.29 0.28 0.26 0.22 0.21 0.2 0.2 0.19 0.19 0.19 0.19 0.19 ]  mu_coulomb_temp_vector=[0.3, 0.28, 0.25]  mu_coulomb_matrix=[0.34, 0.32, 0.3; 0.3, 0.28, 0.25; 0.25, 0.2, 0.15]  mu_interp_method=1  mu_extrap_method=1  d_f=1  w_tol=0.001 rad/s  pressure_min=100 Pa  mu_visc=0 N*m/(rad/s)  initial_state_locked=0  enable_faults=simscape.enum.onoff.off  fault_type=sdl.enum.clutchFault.lock  external_fault=simscape.enum.onoff.off  temporal_fault=simscape.enum.onoff.off  fault_time=5 s  report_fault=simscape.enum.assert.action.none  thermal_mass=25 kJ/K  T_init=300 K
      settings: SourceProductName=Driveline  InternalSimscapePortConfiguration="{\"Bottom\":[],\"Left\":[{\"id\":\"P\",\"label\":\"P\",\"type\":\"input\"},{\"id\":\"B\",\"label\":\"B\",\"type\":\"foundation.mechanical.rotational.rotational\"}],\"Right\":[{\"id\":\"F\",\"label\":\"F\",\"type\":\"foundation.mechanical.rotational.rotational\"}],\"Top\":[]}"
  Damper Axle : fl_lib/Mechanical/Rotational Elements/Rotational Damper  D=0.001 N*m/(rad/s)  w_specify=off  w_priority=High  w=0 rad/s  w_nominal_specify=off  w_nominal_unit=rad/s  w_nominal_value=1  t_specify=off  t_priority=High  t=0 N*m  t_nominal_specify=off  t_nominal_unit=N*m  t_nominal_value=1
      settings: SourceProductName=Foundation Library
  Inertia Output Shaft : fl_lib/Mechanical/Rotational Elements/Inertia  inertia=1 kg*m^2  num_ports=foundation.enum.numPorts2.one  w_specify=off  w_priority=High  w=0 rad/s  w_nominal_specify=off  w_nominal_unit=rad/s  w_nominal_value=1  t_specify=off  t_priority=High  t=0 N*m  t_nominal_specify=off  t_nominal_unit=N*m  t_nominal_value=1
      settings: SourceProductName=Foundation Library
  MRRef Damper Axle : fl_lib/Mechanical/Rotational Elements/Mechanical Rotational Reference
      settings: SourceProductName=Foundation Library
  Sensor Output : Subsystem
      mask Display: disp('SO');
  Brake : PMIOPort  Side=Right
  Shaft : PMIOPort  Port=2  Side=Left
  connections:
  Inertia Output Shaft/LConn1 -- Sensor Output/LConn1 -- Shaft/RConn1
  MRRef Damper Axle/LConn1 -- Damper Axle/RConn1 -- Clutch Brake/LConn2
  Brake/RConn1 -- Clutch Brake/LConn1
  Sensor Output/RConn1 -- Clutch Brake/RConn1 -- Damper Axle/LConn1

== system pdmTransmissionCasing3_new/Shaft/Worn Output Shaft ==
  Clutch Brake : sdl_lib/Clutches/Disk Friction Clutch  geometry_model=1  r_eff=100 mm  d_o=150 mm  d_i=100 mm  nS=4  piston_area=0.001 m^2  unidirectional=0  friction_model=1  mu_w_vector=[ 0 0.1 0.2 0.3 0.4 0.5 1 2 5 10 100 1000 ] rad/s  temperature_TLU=[280.0, 300.0, 320.0] K  mu_static=0.35*2  mu_static_vector=[0.4, 0.38, 0.36]  mu_coulomb=0.3  mu_coulomb_vector=[ 0.29 0.28 0.26 0.22 0.21 0.2 0.2 0.19 0.19 0.19 0.19 0.19 ]  mu_coulomb_temp_vector=[0.3, 0.28, 0.25]  mu_coulomb_matrix=[0.34, 0.32, 0.3; 0.3, 0.28, 0.25; 0.25, 0.2, 0.15]  mu_interp_method=1  mu_extrap_method=1  d_f=1  w_tol=0.001 rad/s  pressure_min=100 Pa  mu_visc=0 N*m/(rad/s)  initial_state_locked=0  enable_faults=simscape.enum.onoff.off  fault_type=sdl.enum.clutchFault.lock  external_fault=simscape.enum.onoff.off  temporal_fault=simscape.enum.onoff.off  fault_time=5 s  report_fault=simscape.enum.assert.action.none  thermal_mass=25 kJ/K  T_init=300 K
      settings: SourceProductName=Driveline  InternalSimscapePortConfiguration="{\"Bottom\":[],\"Left\":[{\"id\":\"P\",\"label\":\"P\",\"type\":\"input\"},{\"id\":\"B\",\"label\":\"B\",\"type\":\"foundation.mechanical.rotational.rotational\"}],\"Right\":[{\"id\":\"F\",\"label\":\"F\",\"type\":\"foundation.mechanical.rotational.rotational\"}],\"Top\":[]}"
  Damper Axle : fl_lib/Mechanical/Rotational Elements/Rotational Damper  D=0.0001 N*m/(rad/s)  w_specify=off  w_priority=High  w=0 rad/s  w_nominal_specify=off  w_nominal_unit=rad/s  w_nominal_value=1  t_specify=off  t_priority=High  t=0 N*m  t_nominal_specify=off  t_nominal_unit=N*m  t_nominal_value=1
      settings: SourceProductName=Foundation Library
  Inertia Output Shaft : fl_lib/Mechanical/Rotational Elements/Inertia  inertia=1 kg*m^2  num_ports=foundation.enum.numPorts2.one  w_specify=off  w_priority=High  w=0 rad/s  w_nominal_specify=off  w_nominal_unit=rad/s  w_nominal_value=1  t_specify=off  t_priority=High  t=0 N*m  t_nominal_specify=off  t_nominal_unit=N*m  t_nominal_value=1
      settings: SourceProductName=Foundation Library
  MRRef Damper Axle : fl_lib/Mechanical/Rotational Elements/Mechanical Rotational Reference
      settings: SourceProductName=Foundation Library
  Sensor Output : Subsystem
      mask Display: disp('SO');
  Brake : PMIOPort  Side=Right
  Shaft : PMIOPort  Port=2  Side=Left
  connections:
  Inertia Output Shaft/LConn1 -- Sensor Output/LConn1 -- Shaft/RConn1
  MRRef Damper Axle/LConn1 -- Damper Axle/RConn1 -- Clutch Brake/LConn2
  Brake/RConn1 -- Clutch Brake/LConn1
  Sensor Output/RConn1 -- Clutch Brake/RConn1 -- Damper Axle/LConn1

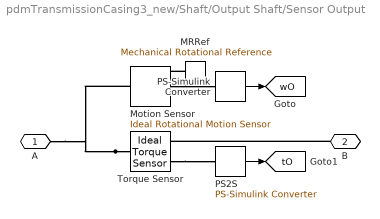
== system pdmTransmissionCasing3_new/Shaft/Output Shaft/Sensor Output ==
  MRRef : fl_lib/Mechanical/Rotational Elements/Mechanical Rotational Reference
      settings: SourceProductName=Foundation Library
  Motion Sensor : fl_lib/Mechanical/Mechanical Sensors/Ideal Rotational Motion Sensor  wrap_angle=simscape.enum.onoff.off  offset=0 rad
      settings: SourceProductName=Foundation Library
  PS-Simulink Converter : nesl_utility/PS-Simulink Converter  PhysicalDomain=network_engine_domain  SubClassName=ps_output  LeftPortType=input  RightPortType=output  PseudoPeriodic=off  Frequencies=[]  Unit=rpm  AffineConversion=off
      settings: SourceProductName=Utilities
  PS2S : nesl_utility/PS-Simulink Converter  PhysicalDomain=network_engine_domain  SubClassName=ps_output  LeftPortType=input  RightPortType=output  PseudoPeriodic=off  Frequencies=[]  Unit=1  AffineConversion=off
      settings: SourceProductName=Utilities
  Torque Sensor : fl_lib/Mechanical/Mechanical Sensors/Ideal Torque Sensor
      settings: SourceProductName=Foundation Library
  A : PMIOPort  Side=Left
  B : PMIOPort  Port=2  Side=Right
  tag scope: tO=global, wO=global
  wires:
  PS2S/1 -> [tO]
  PS-Simulink Converter/1 -> [wO]
  connections:
  Torque Sensor/LConn1 -- A/RConn1 -- Motion Sensor/LConn1
  Motion Sensor/RConn2 -- PS-Simulink Converter/LConn1
  B/RConn1 -- Torque Sensor/RConn1
  MRRef/LConn1 -- Motion Sensor/RConn1
  Torque Sensor/RConn2 -- PS2S/LConn1

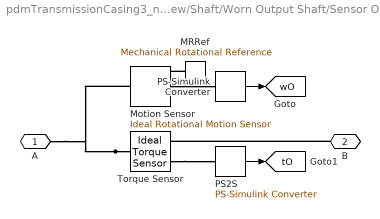
== system pdmTransmissionCasing3_new/Shaft/Worn Output Shaft/Sensor Output ==
  MRRef : fl_lib/Mechanical/Rotational Elements/Mechanical Rotational Reference
      settings: SourceProductName=Foundation Library
  Motion Sensor : fl_lib/Mechanical/Mechanical Sensors/Ideal Rotational Motion Sensor  wrap_angle=simscape.enum.onoff.off  offset=0 rad
      settings: SourceProductName=Foundation Library
  PS-Simulink Converter : nesl_utility/PS-Simulink Converter  PhysicalDomain=network_engine_domain  SubClassName=ps_output  LeftPortType=input  RightPortType=output  PseudoPeriodic=off  Frequencies=[]  Unit=rpm  AffineConversion=off
      settings: SourceProductName=Utilities
  PS2S : nesl_utility/PS-Simulink Converter  PhysicalDomain=network_engine_domain  SubClassName=ps_output  LeftPortType=input  RightPortType=output  PseudoPeriodic=off  Frequencies=[]  Unit=1  AffineConversion=off
      settings: SourceProductName=Utilities
  Torque Sensor : fl_lib/Mechanical/Mechanical Sensors/Ideal Torque Sensor
      settings: SourceProductName=Foundation Library
  A : PMIOPort  Side=Left
  B : PMIOPort  Port=2  Side=Right
  tag scope: tO=global, wO=global
  wires:
  PS2S/1 -> [tO]
  PS-Simulink Converter/1 -> [wO]
  connections:
  Torque Sensor/LConn1 -- A/RConn1 -- Motion Sensor/LConn1
  Motion Sensor/RConn2 -- PS-Simulink Converter/LConn1
  B/RConn1 -- Torque Sensor/RConn1
  MRRef/LConn1 -- Motion Sensor/RConn1
  Torque Sensor/RConn2 -- PS2S/LConn1

== matlab function pdmTransmissionCasing3_new/AMPRBS BRAKE/Amplitude Modulated Pseudo-Random Bit Sequences ==
  data: time input; min_hold_time input; max_hold_time input; min_hold_time_0_brake input; max_hold_time_0_brake input; min_value input; max_value input; int_value input; random_value input; random_value output; random_hold_time input; random_hold_time output; previous_holding_time input; previous_holding_time output
function [random_value, random_hold_time, previous_holding_time]= fcn(time, min_hold_time, max_hold_time, min_hold_time_0_brake, max_hold_time_0_brake, min_value, max_value, int_value, random_value, random_hold_time, previous_holding_time)
%#codegen
if previous_holding_time + random_hold_time <= time
    %zmiana ziarna zeby inne losowanie za kazdym razem bylo
    rng('shuffle')
    %jezeli int_value = 1 to losuj tylko calkowite liczby z zakresu w
    %przeciwnym razie tez niecalkowite
    if int_value == 1 
        random_value = randi([min_value max_value]);
    else
        random_value = (max_value-min_value)*rand(1,1) + min_value;
    end
    if random_value == max_value
        random_hold_time = (max_hold_time_0_brake - min_hold_time_0_brake)*rand(1,1) + min_hold_time_0_brake;
    else
        random_hold_time = (max_hold_time - min_hold_time)*rand(1,1) + min_hold_time;
    end
    previous_holding_time = time;
end
